simulink model "mot_ctrl"  (Simulink 4.00)
settings: Solver=ode45  SolverMode=SingleTasking  StartTime=0.0  StopTime=2  MaxStep=1  RelTol=1e-3  AbsTol=1e-3
values from neighbouring files (symbols this model uses):
  b = 0.1    [MOTOR.M]
  J = 0.01    [MOTOR.M]
  K = 0.01    [MOTOR.M]
  L = 0.5    [MOTOR.M]
  R = 1    [MOTOR.M]
settings Model: LastModifiedBy=R.Babuska  SaveTime=off  SaveOutput=off  LimitDataPoints=off  RTWTemplateMakefile=grt_vc.tmf

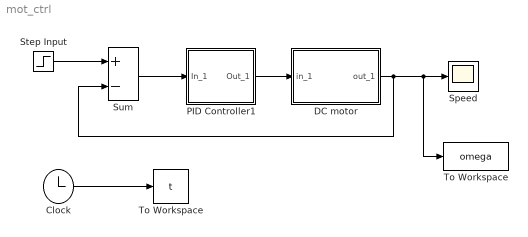
== system mot_ctrl ==
  Clock : Clock
      settings: DisplayTime=off  Decimation=10
  DC motor : Subsystem
      settings: RTWFcnNameOpts=Auto  RTWFileNameOpts=Auto
      mask Display: disp('DC motor')
  PID Controller1 : Subsystem  mask(PID Controller){@1=100, @2=100, @3=10}
      mask prompts: @1 "Proportional:"; @2 "Integral"; @3 "Derivative:"
      mask help:
      | Enter expressions for proportional, integral, and derivative terms.
      | P+I/s+Ds
      mask init:
      | P=@1; I=@2; D=@3;
      settings: RTWFcnNameOpts=Auto  RTWFileNameOpts=Auto
      mask Help: This block implements a PID controller where parameters are entered for the Proportional, Integral and Derivative terms. Unmask this block to see how it works. The derivative term is implemented using a true derivative block.
      mask Display: disp('PID')
  Speed : Scope
      settings: TickLabels=on  TimeRange=auto  YMin=0  YMax=1.5  SaveToWorkspace=off  SaveName=ScopeData  DataFormat=Array  LimitDataPoints=on  MaxDataPoints=5000
  Step Input : Step  Time=0  Before=0  After=1  SampleTime=-1
  Sum : Sum  Inputs=+-  SaturateOnIntegerOverflow=on
  To Workspace : ToWorkspace  VariableName=omega  SampleTime=0  SaveFormat=Array
      settings: MaxDataPoints=1000
  "To Workspace  " : ToWorkspace  VariableName=t  SampleTime=0  SaveFormat=Array
      settings: MaxDataPoints=1000
  wires:
  DC motor/1(out_1) -> Sum/2, To Workspace/1, Speed/1
  Sum/1 -> PID Controller1/1(In_1)
  Step Input/1 -> Sum/1
  PID Controller1/1(Out_1) -> DC motor/1(in_1)
  Clock/1 -> "To Workspace  "/1

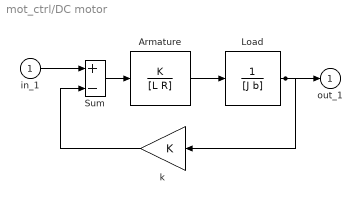
== system mot_ctrl/DC motor ==
  in_1 : Inport  Port=1  LatchInput=off
  " k " : Gain  Orientation=left  Gain=K  Multiplication=Element-wise(K.*u)  SaturateOnIntegerOverflow=on
  Armature : TransferFcn  Numerator=K  Denominator=[L R]  AbsoluteTolerance=auto  Realization=auto
  Load : TransferFcn  Numerator=1  Denominator=[J b]  AbsoluteTolerance=auto  Realization=auto
  Sum : Sum  Inputs=+-  SaturateOnIntegerOverflow=on
  out_1 : Outport  Port=1  InitialOutput=0
  wires:
  Load/1 -> out_1/1, " k "/1
  in_1/1 -> Sum/1
  Sum/1 -> Armature/1
  Armature/1 -> Load/1
  " k "/1 -> Sum/2

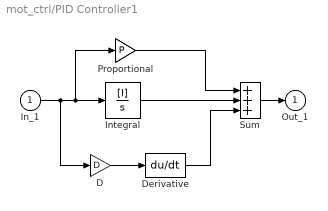
== system mot_ctrl/PID Controller1 ==
  In_1 : Inport  Port=1  LatchInput=off
  D : Gain  Gain=D  Multiplication=Element-wise(K.*u)  SaturateOnIntegerOverflow=on
  Derivative : Derivative
  Integral : TransferFcn  Numerator=[I]  Denominator=[1 0]  AbsoluteTolerance=auto  Realization=auto
  Proportional : Gain  Gain=P  Multiplication=Element-wise(K.*u)  SaturateOnIntegerOverflow=on
  Sum : Sum  Inputs=+++  SaturateOnIntegerOverflow=on
  Out_1 : Outport  Port=1  InitialOutput=0
  wires:
  D/1 -> Derivative/1
  Sum/1 -> Out_1/1
  In_1/1 -> D/1, Proportional/1, Integral/1
  Derivative/1 -> Sum/3
  Integral/1 -> Sum/2
  Proportional/1 -> Sum/1
